simulink model "mrsLidarAndObjectModel"  (R2019a)
settings: Solver=VariableStepAuto  StartTime=0.0  StopTime=10  FixedStep=0.01  RelTol=1e-3  EnableMultiTasking=on
PreLoadFcn:
  | % Simulation parameters
  | load exampleMap
  | sampleTime = 0.05;
  | 
  | % Lidar parameters
  | sensorOffset = [0,0];
  | scanAngles = [-3*pi/8;-pi/4;-pi/8;0;pi/8;pi/4;3*pi/8];
  | maxRange = 6;
  | 
  | % Object Detector parameters
  | objX = 4;
  | objY = 4;
  | targetLabel = 1;
  | objLabel = 1;
  | objDetectorOffset = [0 0];
  | objDetectorAngle = 0;
  | objDetectorFOV = pi/3;
  | objDetectorRange = 5;
  | objDetectorColors = [1 0 0;0 1 0;0 0 1];
  | objDetectorMaxHits = 3;
libraries: mobileRoboticsLib x4
settings Model: EnablePacing=on  Creator=scastro  LastModifiedBy=mejiasal
settings DataIOCC: LimitDataPoints=on  ReturnWorkspaceOutputs=off
settings OptimizationCC: LifeSpan=inf
settings DebuggingCC: AllowSymbolicDim=off  PregeneratedLibrarySubsystemCodeDiagnostic=none  SFUnexpectedBacktrackingDiag=warning  SFNoUnconditionalDefaultTransitionDiag=warning  SFExecutionAtInitializationDiag=none  ArithmeticOperatorsInVariantConditions=warning
settings SFSimCC: SimUseLocalCustomCode=off
settings RTWCC: RTWUseLocalCustomCode=off
settings CodeAppCC: StateflowObjectComments=on
settings GRTTargetCC: TargetLangStandard=C89/C90 (ANSI)  GeneratePreprocessorConditionals=Disable all
settings ConfigComp: CovMetricSettings=dw  CovHtmlReporting=on  CovSaveCumulativeToWorkspaceVar=on  CovSaveSingleToWorkspaceVar=on  CovExternalEMLEnable=off  CovSFcnEnable=off
settings SimscapeCC: SimscapeNominalValues="[{\"value\":\"10\",\"unit\":\"V\"},{\"value\":\"1\",\"unit\":\"A\"},{\"value\":\"10\",\"unit\":\"N*m\"},{\"value\":\"10\",\"unit\":\"bar\"},{\"value\":\"100\",\"unit\":\"kJ/kg\"},{\"value\":\"1\",\"unit\":\"kW\"},{\"value\":\"300\",\"unit\":\"K\"},{\"value\":\"100\",\"unit\":\"cm^3/s\"},{\"value\":\"1\",\"unit\":\"kN\"},{\"value\":\"1\",\"unit\":\"g/cm^3\"},{\"value\":\"1\",\"unit\":\"l\"},{\"value\":\"1\",\"unit\":\"cm^2\"},{\"value\":\"60\",\"unit\":\"Hz\"}]"  SimscapeLogType=all  SimscapeLogDataHistory=10000
settings ConfigurationSet: Description=SimMechanics 2G
settings ExplorerConfigSet: InternalSimMechanicsExplorerSettings="<ExplorerConfiguration><canonicalview>default</canonicalview><AnimationSetting><BasePlaybackSpeed>1.0</BasePlaybackSpeed><PlaybackSpeedFactor>1.0</PlaybackSpeedFactor></AnimationSetting><TilePanel><TileInfo><Tiles Columns=\"1\" Count=\"1\" Rows=\"1\"><Column Weight=\"1\"/><Row Weight=\"1\"/><Tile Height=\"1\" Width=\"1\" X=\"0\" Y=\"0\"/></Tiles></TileInfo><SceneInfo><SceneViewer><BGColor><R>0.60000002384185791</R><G>0.60000002384185791</G><B>0.60000002384185791</B></BGColor><Camera><DoPerspective>off</DoPerspective><Position><X>-1.70656042355848525</X><Y>-0.974920623359631922</Y><Z>4.72930454537082046</Z></Position><Center><X>0.552860638431633689</X><Y>1.42025063411503494</Y><Z>1.4843509506914252</Z></Center><Up><X>0.664249622453917166</X><Y>0.300615402055903091</Y><Z>0.684399604848363485</Z></Up><ViewLimDist>1</ViewLimDist><YLim>2.77881717169207398</YLim><XLim>3.55928742670435394</XLim></Camera></SceneViewer></SceneInfo></TilePanel><MechEditorPanel><Cameras/><GfxPanelCameraMap/><VideoCreator><PlaybackSpeedRatio>1.0</PlaybackSpeedRatio><FrameRate>30</FrameRate><VideoFormat>Motion JPEG AVI</VideoFormat><FrameSize>auto</FrameSize></VideoCreator></MechEditorPanel></ExplorerConfiguration>"

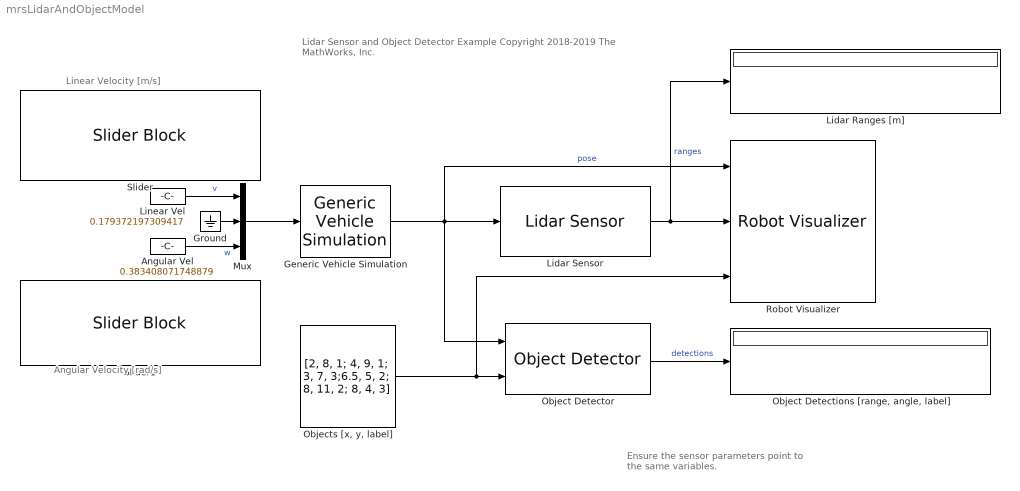
== system mrsLidarAndObjectModel ==
  note: Linear Velocity [m/s]
  note: Angular Velocity [rad/s]
  note: Lidar Sensor and Object Detector Example
      |
      | Copyright 2018-2019 The MathWorks, Inc.
  note: Ensure the sensor parameters point to the same variables.
  Angular Vel : Constant  Value=0.383408071748879
  Generic Vehicle Simulation : mobileRoboticsLib/Utilities/Generic Vehicle Simulation  initX=6  initY=8  initAngle=0  Ts=sampleTime
      settings: SourceProductName=Mobile Robotics Simulation Library
  Ground : Ground
  Lidar Ranges [m] : Display
  Lidar Sensor : mobileRoboticsLib/Environments/Lidar Sensor  mapName=map  sensorOffset=sensorOffset  scanAngles=scanAngles  maxRange=maxRange
      settings: SourceProductName=Ground Vehicles Library
  Linear Vel : Constant  Value=0.179372197309417
  Mux : Mux  Inputs=3
  "Object Detections [range, angle, label]" : Display
  Object Detector : mobileRoboticsLib/Environments/Object Detector  mapName=map  sensorOffset=objDetectorOffset  sensorAngle=objDetectorAngle  fieldOfView=objDetectorFOV  maxRange=objDetectorRange  maxDetections=objDetectorMaxHits  sampleTime=0.1
      settings: SourceProductName=Ground Vehicles Library
  "Objects [x, y, label]" : Constant  Value=[2, 8, 1; 4, 9, 1; 3, 7, 3;6.5, 5, 2; 8, 11, 2; 8, 4, 3]
  Robot Visualizer : mobileRoboticsLib/Environments/Robot Visualizer  Priority=99  robotRadius=0  mapName=map  showTrajectory=off  hasWaypoints=off  hasLidar=on  sensorOffset=sensorOffset  scanAngles=scanAngles  hasObjDetector=on  objDetectorOffset=objDetectorOffset  objDetectorAngle=objDetectorAngle  objDetectorFOV=objDetectorFOV  objDetectorMaxRange=objDetectorRange  objectColors=objDetectorColors  objectMarkers=s
      settings: SourceProductName=Ground Vehicles Library
  Slider : SliderBlock  ScaleMax=1
  Slider1 : SliderBlock  ScaleMin=-1.5  ScaleMax=1.5
  wires:
  Generic Vehicle Simulation/1 -> Lidar Sensor/1, Robot Visualizer/1, Object Detector/1  "pose"
  Angular Vel/1 -> Mux/3  "w"
  Mux/1 -> Generic Vehicle Simulation/1
  Linear Vel/1 -> Mux/1  "v"
  Ground/1 -> Mux/2
  "Objects [x, y, label]"/1 -> Robot Visualizer/3, Object Detector/2
  Object Detector/1 -> "Object Detections [range, angle, label]"/1  "detections"
  Lidar Sensor/1 -> Lidar Ranges [m]/1, Robot Visualizer/2  "ranges"
